simulink library "CockpitDisplayLib"  (R2013b)
settings: Solver=ode45  StartTime=0.0  StopTime=10.0  RelTol=1e-3
undefined symbols (not defined in the file): Ts
libraries: dspadpt3 x3, sf_aircraft_screen_library x1, LandingGearModeLib x1
(part 1 of 2)
settings Model: Creator=siddhars  LastModifiedBy=siddhars

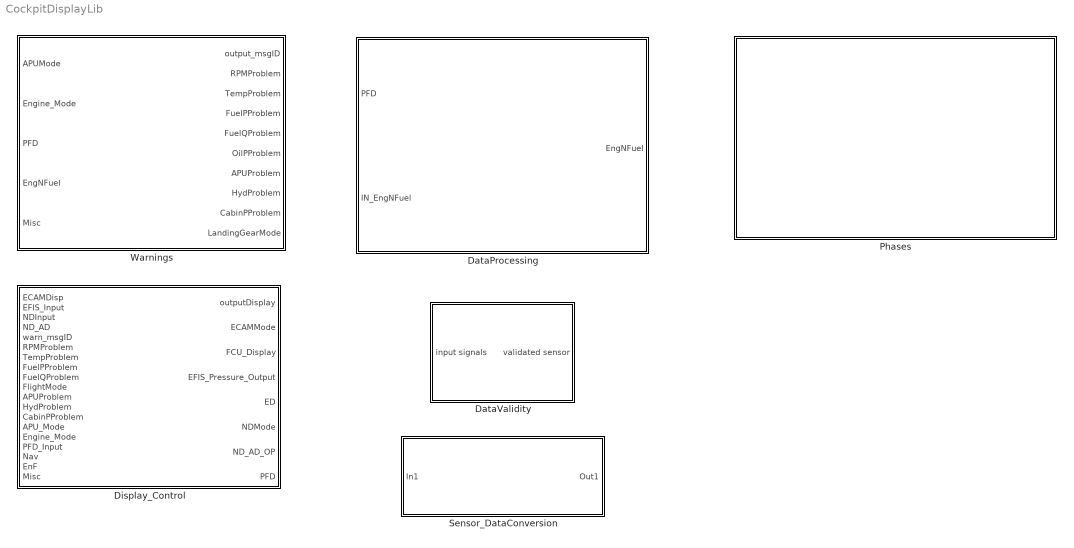
== system CockpitDisplayLib ==
  DataProcessing : Stateflow chart  TreatAsAtomicUnit=on
  DataValidity : Subsystem
  Display_Control : Stateflow chart  TreatAsAtomicUnit=on
  Phases : Stateflow chart  TreatAsAtomicUnit=on
  Sensor_DataConversion : Subsystem  mask{noise_factor=1}
      mask prompts: noise_factor "noise factor"
      mask Callback noise_factor: noise_factor = 1;
  Warnings : Stateflow chart  Priority=0  TreatAsAtomicUnit=on

== system CockpitDisplayLib/DataProcessing/RPMCalc.signal_conditioning ==
  RPM : Inport  OutDataTypeStr=double  PortDimensions=[3 1]
  f : TriggerPort  TriggerType=function-call
      settings: CopyFcn=Stateflow.SLINSF.SimulinkMan.removeBlockPreDeleteFcn  PreDeleteFcn=Stateflow.SLINSF.SimulinkMan.unsafePredeleteFcn
  DataValidity : sf_aircraft_screen_library/Position Monitor, (No Filter)
  Out : Outport
  wires:
  DataValidity/1 -> Out/1
  RPM/1 -> DataValidity/1

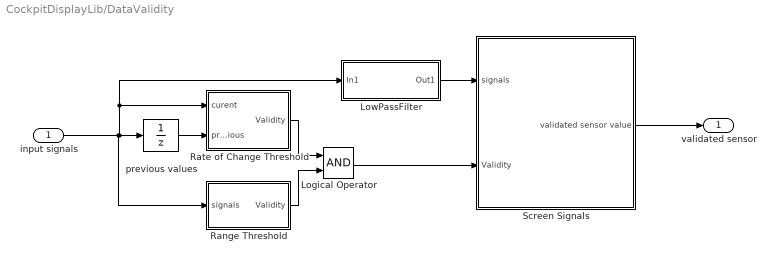
== system CockpitDisplayLib/DataValidity ==
  input signals : Inport  PortDimensions=3
  Logical Operator : Logic  AllPortsSameDT=off
  LowPassFilter : Subsystem
  Range Threshold : Subsystem  RequirementInfo={'other' 'Position Sensor Logic Requirements.doc' 'Out of Bound Readings' 'true' 'Out of Bound Readings' '' } %GIDa_9464ebc1_75a4_4fc1_b22e_333f2b8b1e7f
  Rate of Change Threshold : Subsystem  RequirementInfo={'other' 'Position Sensor Logic Requirements.doc' 'Rate of Change of Readings' 'true' 'Rate of Change of Readings' '' } %GIDa_c48669ac_f48f_472f_ad85_0df61b6d7184  mask{max_rate_change=20000}
      mask prompts: max_rate_change "Rate Change Threshold"
  Screen Signals : Subsystem
  previous values : UnitDelay  SampleTime=-1
  validated sensor : Outport
  wires:
  LowPassFilter/1(Out1) -> Screen Signals/1(signals)
  Screen Signals/1(validated sensor value) -> validated sensor/1
  input signals/1 -> Range Threshold/1(signals), previous values/1, Rate of Change Threshold/1(curent), LowPassFilter/1(In1)
  previous values/1 -> Rate of Change Threshold/2(previous)
  Range Threshold/1(Validity) -> Logical Operator/2
  Rate of Change Threshold/1(Validity) -> Logical Operator/1
  Logical Operator/1 -> Screen Signals/2(Validity)

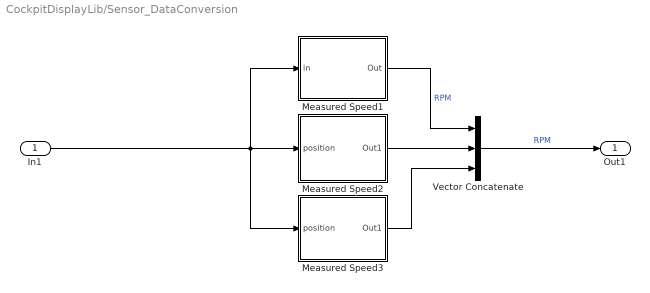
== system CockpitDisplayLib/Sensor_DataConversion ==
  In1 : Inport
  Measured Speed1 : Subsystem
  Measured Speed2 : Subsystem
  Measured Speed3 : Subsystem
  Vector Concatenate : Concatenate  NumInputs=3
  Out1 : Outport
  wires:
  Measured Speed1/1(Out) -> Vector Concatenate/1  "RPM"
  Vector Concatenate/1 -> Out1/1  "RPM"
  Measured Speed3/1(Out1) -> Vector Concatenate/3
  In1/1 -> Measured Speed3/1(position), Measured Speed1/1(in), Measured Speed2/1(position)
  Measured Speed2/1(Out1) -> Vector Concatenate/2

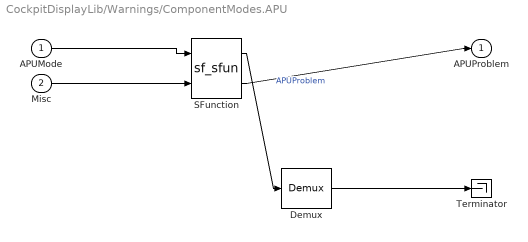
== system CockpitDisplayLib/Warnings/ComponentModes.APU ==
  APUMode : Inport
  Misc : Inport  Port=2
  " Demux " : Demux  Outputs=1
  " SFunction " : S-Function  Tag=Stateflow S-Function CockpitDisplayLib 10  FunctionName=sf_sfun  PortCounts=[2 2]  EnableBusSupport=off
  " Terminator " : Terminator
  APUProblem : Outport
  wires:
  APUMode/1 -> " SFunction "/1
  Misc/1 -> " SFunction "/2
  " SFunction "/2 -> APUProblem/1  "APUProblem"
  " Demux "/1 -> " Terminator "/1
  " SFunction "/1 -> " Demux "/1

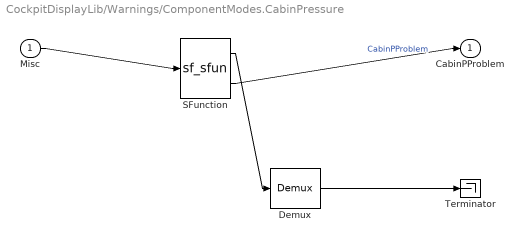
== system CockpitDisplayLib/Warnings/ComponentModes.CabinPressure ==
  Misc : Inport
  " Demux " : Demux  Outputs=1
  " SFunction " : S-Function  Tag=Stateflow S-Function CockpitDisplayLib 11  FunctionName=sf_sfun  PortCounts=[1 2]  EnableBusSupport=off
  " Terminator " : Terminator
  CabinPProblem : Outport
  wires:
  Misc/1 -> " SFunction "/1
  " SFunction "/2 -> CabinPProblem/1  "CabinPProblem"
  " Demux "/1 -> " Terminator "/1
  " SFunction "/1 -> " Demux "/1

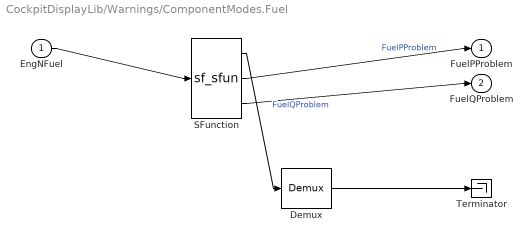
== system CockpitDisplayLib/Warnings/ComponentModes.Fuel ==
  EngNFuel : Inport
  " Demux " : Demux  Outputs=1
  " SFunction " : S-Function  Tag=Stateflow S-Function CockpitDisplayLib 2  FunctionName=sf_sfun  PortCounts=[1 3]  EnableBusSupport=off
  " Terminator " : Terminator
  FuelPProblem : Outport
  FuelQProblem : Outport  Port=2
  wires:
  EngNFuel/1 -> " SFunction "/1
  " SFunction "/2 -> FuelPProblem/1  "FuelPProblem"
  " SFunction "/3 -> FuelQProblem/1  "FuelQProblem"
  " Demux "/1 -> " Terminator "/1
  " SFunction "/1 -> " Demux "/1

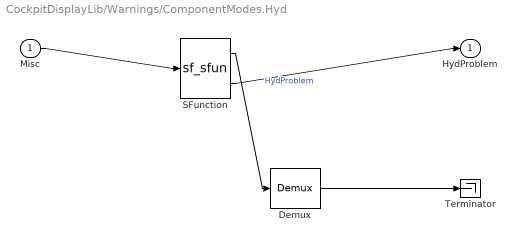
== system CockpitDisplayLib/Warnings/ComponentModes.Hyd ==
  Misc : Inport
  " Demux " : Demux  Outputs=1
  " SFunction " : S-Function  Tag=Stateflow S-Function CockpitDisplayLib 13  FunctionName=sf_sfun  PortCounts=[1 2]  EnableBusSupport=off
  " Terminator " : Terminator
  HydProblem : Outport
  wires:
  Misc/1 -> " SFunction "/1
  " SFunction "/2 -> HydProblem/1  "HydProblem"
  " Demux "/1 -> " Terminator "/1
  " SFunction "/1 -> " Demux "/1

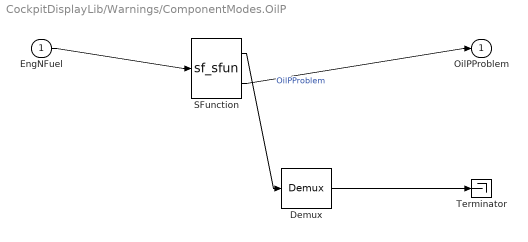
== system CockpitDisplayLib/Warnings/ComponentModes.OilP ==
  EngNFuel : Inport
  " Demux " : Demux  Outputs=1
  " SFunction " : S-Function  Tag=Stateflow S-Function CockpitDisplayLib 15  FunctionName=sf_sfun  PortCounts=[1 2]  EnableBusSupport=off
  " Terminator " : Terminator
  OilPProblem : Outport
  wires:
  EngNFuel/1 -> " SFunction "/1
  " SFunction "/2 -> OilPProblem/1  "OilPProblem"
  " Demux "/1 -> " Terminator "/1
  " SFunction "/1 -> " Demux "/1

== system CockpitDisplayLib/Warnings/ComponentModes.RPM ==
  EngNFuel : Inport
  " Demux " : Demux  Outputs=1
  " SFunction " : S-Function  Tag=Stateflow S-Function CockpitDisplayLib 16  FunctionName=sf_sfun  PortCounts=[1 2]  EnableBusSupport=off
  " Terminator " : Terminator
  RPMProblem : Outport
  wires:
  EngNFuel/1 -> " SFunction "/1
  " SFunction "/2 -> RPMProblem/1  "RPMProblem"
  " Demux "/1 -> " Terminator "/1
  " SFunction "/1 -> " Demux "/1

== system CockpitDisplayLib/Warnings/ComponentModes.Temp ==
  EngNFuel : Inport
  " Demux " : Demux  Outputs=1
  " SFunction " : S-Function  Tag=Stateflow S-Function CockpitDisplayLib 17  FunctionName=sf_sfun  PortCounts=[1 2]  EnableBusSupport=off
  " Terminator " : Terminator
  TempProblem : Outport
  wires:
  EngNFuel/1 -> " SFunction "/1
  " SFunction "/2 -> TempProblem/1  "TempProblem"
  " Demux "/1 -> " Terminator "/1
  " SFunction "/1 -> " Demux "/1

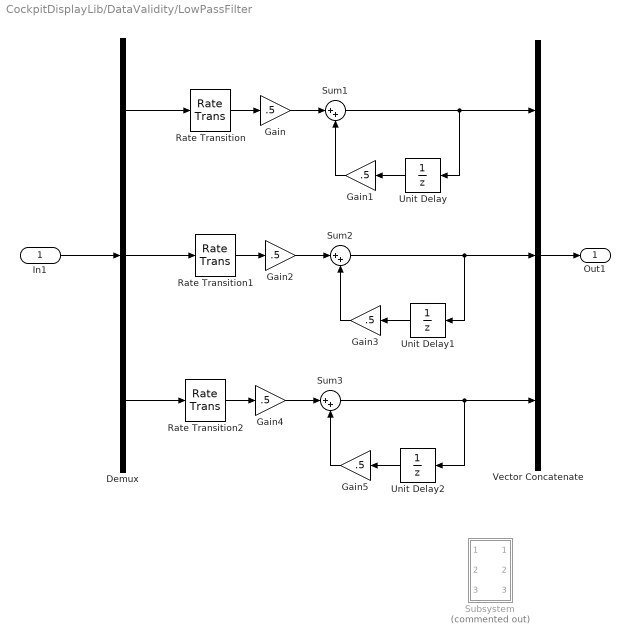
== system CockpitDisplayLib/DataValidity/LowPassFilter ==
  In1 : Inport
  Demux : Demux  Outputs=3
  Gain{,1..5} (6 alike) : Gain  Gain=.5
  Rate Transition : RateTransition
  Rate Transition1 : RateTransition
  Rate Transition2 : RateTransition
  Subsystem : Subsystem  Commented=on
  Sum1 : Sum  Inputs=|++
  Sum2 : Sum  Inputs=|++
  Sum3 : Sum  Inputs=|++
  Unit Delay : UnitDelay  SampleTime=-1
  Unit Delay1 : UnitDelay  SampleTime=-1
  Unit Delay2 : UnitDelay  SampleTime=-1
  Vector Concatenate : Concatenate  NumInputs=3
  Out1 : Outport
  wires:
  Rate Transition2/1 -> Gain4/1
  Gain5/1 -> Sum3/2
  Unit Delay2/1 -> Gain5/1
  Gain4/1 -> Sum3/1
  Demux/3 -> Rate Transition2/1
  Sum3/1 -> Unit Delay2/1, Vector Concatenate/3
  Rate Transition1/1 -> Gain2/1
  Gain3/1 -> Sum2/2
  Unit Delay1/1 -> Gain3/1
  Gain2/1 -> Sum2/1
  Demux/2 -> Rate Transition1/1
  Sum2/1 -> Unit Delay1/1, Vector Concatenate/2
  Rate Transition/1 -> Gain/1
  Gain1/1 -> Sum1/2
  Unit Delay/1 -> Gain1/1
  Gain/1 -> Sum1/1
  Demux/1 -> Rate Transition/1
  Sum1/1 -> Vector Concatenate/1, Unit Delay/1
  In1/1 -> Demux/1
  Vector Concatenate/1 -> Out1/1

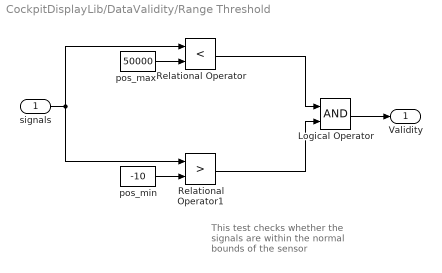
== system CockpitDisplayLib/DataValidity/Range Threshold ==
  note: This test checks whether the signals are within
      | the normal bounds of the sensor
  signals : Inport
  Logical Operator : Logic  AllPortsSameDT=off
  Relational Operator : RelationalOperator  Operator=<
  Relational Operator1 : RelationalOperator  Operator=>
  pos_max : Constant  Value=50000
  pos_min : Constant  Value=-10
  Validity : Outport
  wires:
  Logical Operator/1 -> Validity/1
  pos_min/1 -> Relational Operator1/2
  pos_max/1 -> Relational Operator/2
  Relational Operator1/1 -> Logical Operator/2
  Relational Operator/1 -> Logical Operator/1
  signals/1 -> Relational Operator1/1, Relational Operator/1

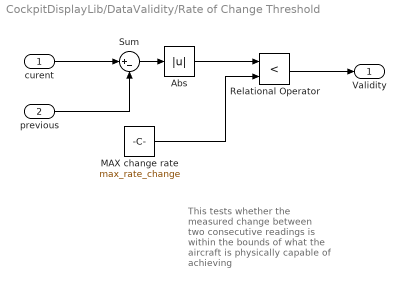
== system CockpitDisplayLib/DataValidity/Rate of Change Threshold ==
  note: This tests whether the measured change between two consecutive readings
      | is within the bounds of what the aircraft is physically capable of achieving
  curent : Inport
  previous : Inport  Port=2
  Abs : Abs  SaturateOnIntegerOverflow=on
  MAX change rate : Constant  Value=max_rate_change
  Relational Operator : RelationalOperator  Operator=<  OutDataTypeStr=boolean
  Sum : Sum  Inputs=|+-  SaturateOnIntegerOverflow=on
  Validity : Outport
  wires:
  curent/1 -> Sum/1
  previous/1 -> Sum/2
  Relational Operator/1 -> Validity/1
  MAX change rate/1 -> Relational Operator/2
  Sum/1 -> Abs/1
  Abs/1 -> Relational Operator/1

== system CockpitDisplayLib/DataValidity/Screen Signals ==
  signals : Inport
  Validity : Inport  Port=2
  Chart (MATLAB) : Stateflow chart  TreatAsAtomicUnit=on
  Data Type Conversion : DataTypeConversion  OutDataTypeStr=double
  validated sensor value : Outport
  wires:
  Chart (MATLAB)/1(valid_signal) -> validated sensor value/1
  Validity/1 -> Data Type Conversion/1
  signals/1 -> Chart (MATLAB)/1(signals)
  Data Type Conversion/1 -> Chart (MATLAB)/2(validity)

== system CockpitDisplayLib/Sensor_DataConversion/Measured Speed1 ==
  in : Inport
  Random Number : RandomNumber  Variance=.001*noise_factor  SampleTime=Ts
  Sum1 : Sum  Inputs=|++  SaturateOnIntegerOverflow=on
  Out : Outport
  wires:
  Sum1/1 -> Out/1
  in/1 -> Sum1/1
  Random Number/1 -> Sum1/2

== system CockpitDisplayLib/Sensor_DataConversion/Measured Speed2 ==
  position : Inport
  Random Number : RandomNumber  Variance=.001*noise_factor  SampleTime=Ts
  Sum1 : Sum  Inputs=|++  SaturateOnIntegerOverflow=on
  Out1 : Outport
  wires:
  Random Number/1 -> Sum1/2
  position/1 -> Sum1/1
  Sum1/1 -> Out1/1

== system CockpitDisplayLib/Sensor_DataConversion/Measured Speed3 ==
  position : Inport
  Random Number : RandomNumber  Variance=.001*noise_factor  SampleTime=Ts
  Sum : Sum  Inputs=|++  SaturateOnIntegerOverflow=on
  Out1 : Outport
  wires:
  Sum/1 -> Out1/1
  position/1 -> Sum/1
  Random Number/1 -> Sum/2

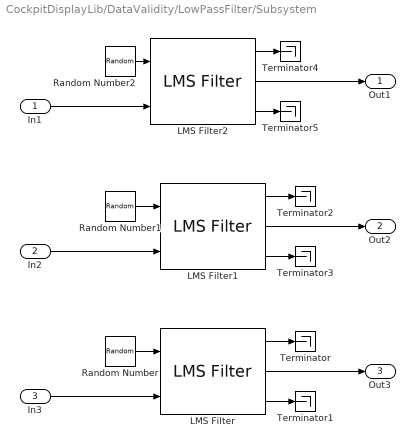
== system CockpitDisplayLib/DataValidity/LowPassFilter/Subsystem ==
  In1 : Inport
  In2 : Inport  Port=2
  In3 : Inport  Port=3
  LMS Filter : dspadpt3/LMS Filter  Algo=LMS  L=2  stepflag=Dialog  mu=0.1  leakage=1.0  ic=0  Adapt=off  resetflag=None  weights=on  secondCoeffMode=User-defined  secondCoeffWordLength=2  secondCoeffFracLength=15  accum2Mode=User-defined  accum2FracLength=20  prodOutput2Mode=User-defined  prodOutput2FracLength=20  prodOutput3Mode=User-defined  prodOutput3FracLength=20  prodOutput4Mode=User-defined  prodOutput4FracLength=20  quotientMode=User-defined  quotientFracLength=20  roundingMode=Floor  overflowMode=off  addnparflag=off
  LMS Filter1 : dspadpt3/LMS Filter  Algo=LMS  L=2  stepflag=Dialog  mu=0.1  leakage=1.0  ic=0  Adapt=off  resetflag=None  weights=on  secondCoeffMode=User-defined  secondCoeffWordLength=2  secondCoeffFracLength=15  accum2Mode=User-defined  accum2FracLength=20  prodOutput2Mode=User-defined  prodOutput2FracLength=20  prodOutput3Mode=User-defined  prodOutput3FracLength=20  prodOutput4Mode=User-defined  prodOutput4FracLength=20  quotientMode=User-defined  quotientFracLength=20  roundingMode=Floor  overflowMode=off  addnparflag=off
  LMS Filter2 : dspadpt3/LMS Filter  Algo=LMS  L=2  stepflag=Dialog  mu=0.1  leakage=1.0  ic=0  Adapt=off  resetflag=None  weights=on  secondCoeffMode=User-defined  secondCoeffWordLength=2  secondCoeffFracLength=15  accum2Mode=User-defined  accum2FracLength=20  prodOutput2Mode=User-defined  prodOutput2FracLength=20  prodOutput3Mode=User-defined  prodOutput3FracLength=20  prodOutput4Mode=User-defined  prodOutput4FracLength=20  quotientMode=User-defined  quotientFracLength=20  roundingMode=Floor  overflowMode=off  addnparflag=off
  Random Number : RandomNumber  Variance=0.01  SampleTime=Ts
  Random Number1 : RandomNumber  Variance=0.01  SampleTime=Ts
  Random Number2 : RandomNumber  Variance=0.01  SampleTime=Ts
  Terminator{,1..5} (6 alike) : Terminator
  Out1 : Outport
  Out2 : Outport  Port=2
  Out3 : Outport  Port=3
  wires:
  LMS Filter2/1 -> Terminator4/1
  LMS Filter2/3 -> Terminator5/1
  Random Number2/1 -> LMS Filter2/1
  LMS Filter1/1 -> Terminator2/1
  Random Number1/1 -> LMS Filter1/1
  LMS Filter/3 -> Terminator1/1
  LMS Filter1/3 -> Terminator3/1
  LMS Filter/2 -> Out3/1
  LMS Filter2/2 -> Out1/1
  In1/1 -> LMS Filter2/2
  In3/1 -> LMS Filter/2
  In2/1 -> LMS Filter1/2
  LMS Filter1/2 -> Out2/1
  Random Number/1 -> LMS Filter/1
  LMS Filter/1 -> Terminator/1

== stateflow chart CockpitDisplayLib/Display_Control ==
  state PrimaryFlightDisplay [parallel]
    entry, during:
    PFD.AirSpeed = PFD_Input.AirSpeed;
    PFD.Attitude = PFD_Input.Attitude;
    PFD.Heading = PFD_Input.Direction;
    PFD.Altitude = PFD_Input.Altitude;
    settings: executionOrder=1
    state AirSpeed [parallel]
      settings: executionOrder=1
      state Starting
        entry:
        PFD.AirSpeedMode = -1;
      state OFF
      state Running
        entry: PFD.AirSpeedMode = 1;
      (default) -> PrimaryFlightDisplay.AirSpeed.OFF
      PrimaryFlightDisplay.AirSpeed.OFF -> PrimaryFlightDisplay.AirSpeed.Starting : [APU_Mode  == 1]
      PrimaryFlightDisplay.AirSpeed.Starting -> PrimaryFlightDisplay.AirSpeed.Running : after(5,sec)
    state Altitude [parallel]
      settings: executionOrder=2
      state OFF
      state Starting
        entry:
        PFD.AltMode = -1;
      state Running
        entry: PFD.AltMode = 1;
      (default) -> PrimaryFlightDisplay.Altitude.OFF
      PrimaryFlightDisplay.Altitude.OFF -> PrimaryFlightDisplay.Altitude.Starting : [APU_Mode  == 1]
      PrimaryFlightDisplay.Altitude.Starting -> PrimaryFlightDisplay.Altitude.Running : after(5,sec)
    state Heading [parallel]
      settings: executionOrder=3
      state OFF
      state Starting
        entry:
        PFD.HeadingMode = -1;
      state Running
        entry: PFD.HeadingMode = 1;
      (default) -> PrimaryFlightDisplay.Heading.OFF
      PrimaryFlightDisplay.Heading.OFF -> PrimaryFlightDisplay.Heading.Starting : [APU_Mode  == 1]
      PrimaryFlightDisplay.Heading.Starting -> PrimaryFlightDisplay.Heading.Running : after(5,sec)
    state Attitude [parallel]
      settings: executionOrder=4
      state OFF
      state Starting
        entry:
        PFD.AttMode = -1;
      state Running
        entry: PFD.AttMode = 1;
      (default) -> PrimaryFlightDisplay.Attitude.OFF
      PrimaryFlightDisplay.Attitude.OFF -> PrimaryFlightDisplay.Attitude.Starting : [APU_Mode  == 1]
      PrimaryFlightDisplay.Attitude.Starting -> PrimaryFlightDisplay.Attitude.Running : after(5,sec)
  state NavigationDisplay [parallel]
    settings: executionOrder=2
    state NDDisplayPages [parallel]
      settings: executionOrder=1
      state NDRunning
        state ILSPage
          entry:
          NDMode = 1;
        state VORPage
          entry:
          NDMode = 2;
        state NAVPage
          entry:
          NDMode = 3;
        state ARCPage
          entry:
          NDMode = 4;
        state PLANPage
          entry:
          NDMode = 5;
        NDRunning -> (junction 257)
        (junction 257) -> ILSPage [order 1] : [NDInput == NDPageInput.ILS]
        (junction 257) -> PLANPage [order 5] : [NDInput == NDPageInput.PLAN]
        (junction 257) -> VORPage [order 2] : [NDInput == NDPageInput.VOR]
        (junction 257) -> ARCPage [order 4] : [NDInput == NDPageInput.ARC]
        (junction 257) -> NAVPage [order 3] : [NDInput == NDPageInput.NAV]
      state NDOff
      state NDStart
        entry:
        NDMode = -1;
      (default) -> NDOff
      NDOff -> NDStart : [APU_Mode  == 1]
      NDStart -> ILSPage : after(3,sec)
    state CSTRDisplay [parallel]
      settings: executionOrder=2
      state OFF
        entry:
        ND_AD_OP.CSTR=0;
      state ON
        entry:
        ND_AD_OP.CSTR=1;
      (default) -> NavigationDisplay.CSTRDisplay.OFF
      NavigationDisplay.CSTRDisplay.OFF -> NavigationDisplay.CSTRDisplay.ON : [ND_AD.CSTR==1&& in(NDDisplayPages.NDRunning)]
      NavigationDisplay.CSTRDisplay.ON -> NavigationDisplay.CSTRDisplay.OFF : [ND_AD.CSTR==0]
    state WPTDisplay [parallel]
      settings: executionOrder=3
      state OFF
        entry:
        ND_AD_OP.WPT=0;
      state ON
        entry:
        ND_AD_OP.WPT=1;
      (default) -> NavigationDisplay.WPTDisplay.OFF
      NavigationDisplay.WPTDisplay.OFF -> NavigationDisplay.WPTDisplay.ON : [ND_AD.WPT==1&& in(NDDisplayPages.NDRunning)]
      NavigationDisplay.WPTDisplay.ON -> NavigationDisplay.WPTDisplay.OFF : [ND_AD.WPT==0]
    state VORDDisplay [parallel]
      settings: executionOrder=4
      state OFF
        entry:
        ND_AD_OP.VORD= 0;
      state ON
        entry:
        ND_AD_OP.VORD= 1;
      (default) -> NavigationDisplay.VORDDisplay.OFF
      NavigationDisplay.VORDDisplay.OFF -> NavigationDisplay.VORDDisplay.ON : [ND_AD.VORD==1&& in(NDDisplayPages.NDRunning)]
      NavigationDisplay.VORDDisplay.ON -> NavigationDisplay.VORDDisplay.OFF : [ND_AD.VORD==0]
    state NDBDisplay [parallel]
      settings: executionOrder=5
      state OFF
        entry:
        ND_AD_OP.NDB= 0;
      state ON
        entry:
        ND_AD_OP.NDB= 1;
      (default) -> NavigationDisplay.NDBDisplay.OFF
      NavigationDisplay.NDBDisplay.OFF -> NavigationDisplay.NDBDisplay.ON : [ND_AD.NDB==1&& in(NDDisplayPages.NDRunning)]
      NavigationDisplay.NDBDisplay.ON -> NavigationDisplay.NDBDisplay.OFF : [ND_AD.NDB==0]
    state ARPTDisplay [parallel]
      settings: executionOrder=6
      state OFF
        entry:
        ND_AD_OP.ARPT= 0;
      state ON
        entry:
        ND_AD_OP.ARPT= 1;
      (default) -> NavigationDisplay.ARPTDisplay.OFF
      NavigationDisplay.ARPTDisplay.OFF -> NavigationDisplay.ARPTDisplay.ON : [ND_AD.ARPT==1&& in(NDDisplayPages.NDRunning)]
      NavigationDisplay.ARPTDisplay.ON -> NavigationDisplay.ARPTDisplay.OFF : [ND_AD.ARPT==0]
  state EngineDisplay [parallel]
    entry, during:
    outputDisplay.warn_msgID = warn_msgID;
    outputDisplay.flightmode = FlightMode;
    ED.N1_L = EnF.RPM;
    ED.N1_R = EnF.RPM;
    ED.FlapConfig = calcFlapConfig(FlightMode);
    ED.EGT1 = EnF.EGT;
    ED.EGT2 = EnF.EGT;
    ED.EPR1 = EnF.EPR1;
    ED.EPR2 = EnF.EPR2;
    ED.FuelQuantity = EnF.FuelQuantity;
    settings: executionOrder=3
    state out = calcFlapConfig(flightphase) [function]
      (default) -> (junction 230) : % comment
      (junction 230) -> (junction 233) [order 1] : [flightphase == 1]
      (junction 230) -> (junction 232) [order 2]
      (junction 233) -> (junction 234) : {out = 1;}
      (junction 232) -> (junction 235) [order 1] : [flightphase == 2]
      (junction 232) -> (junction 231) [order 2] : {out = 3;}
      (junction 235) -> (junction 236) : {out = 2;}
      (junction 236) -> (junction 231)
      (junction 234) -> (junction 236)
      (junction 231) -> (junction 237)
    state Engine_Running
      entry, during:
      ED.ED_Mode_L = 1;
      ED.ED_Mode_R = 1;
      outputDisplay.ED_Mode_L = 1;
      outputDisplay.ED_Mode_R = 1;
    state Engine_Ready
      entry, during:
      ED.ED_Mode_L = 1;
      ED.ED_Mode_R = 1;
      outputDisplay.ED_Mode_L = 1;
      outputDisplay.ED_Mode_R = 1;
    state Engine_Off
    state Engine_Boot
      entry, during:
      ED.ED_Mode_L = -1;
      ED.ED_Mode_R = -1;
      outputDisplay.ED_Mode_L = -1;
      outputDisplay.ED_Mode_R = -1;
    (default) -> Engine_Off
    Engine_Ready -> Engine_Running : [Engine_Mode == 2]
    Engine_Boot -> Engine_Ready : after(5,sec)
    Engine_Off -> Engine_Boot : [Engine_Mode == 1]
  state FCU_EFIS_Display [parallel]
    entry, during:
    FCU_Display.Speed =  PFD_Input.AirSpeed;
    FCU_Display.Heading = Nav.selectedheading;
    FCU_Display.Altitude = PFD_Input.Altitude;
    if EFIS_Input == EFIS_Pressure.inHg
    EFIS_Pressure_Output = Misc.CabinPressure;
    else
    EFIS_Pressure_Output = Misc.CabinPressure*25.4;
    end
    settings: executionOrder=5
  state SystemDisplay [parallel]
    settings: executionOrder=4
    state Startup
      state APU_Ready
        entry:
        ECAMMode = 8;
      state APU_Running
        entry:
        ECAMMode = 8;
      state APU_Boot
        entry:
        ECAMMode = -1;
      state APU_Off
      state APU_Wait
        entry:
        ECAMMode = 11 ;
      state EngineStarting
        entry:
        ECAMMode = 4 ;
      (default) -> APU_Off
      APU_Off -> APU_Boot : [APU_Mode  == 1]
      APU_Boot -> APU_Ready : after(2,sec)
      APU_Ready -> APU_Running : [APU_Mode == 2]
      APU_Wait -> EngineStarting : [Engine_Mode == 1]
      APU_Running -> APU_Wait : after(3,sec)
    state NormalFlight
      state PushbackAndTaxi
        entry: ECAMMode = 1;
      state TakeoffCruiseDescent
        entry: ECAMMode = 2;
      state Land
        entry: ECAMMode = 3;
      NormalFlight -> (junction 92) [order 1]
      (default) -> (junction 92)
      (junction 92) -> PushbackAndTaxi [order 1] : [FlightMode == 1]
      (junction 92) -> Land [order 3]
      (junction 92) -> TakeoffCruiseDescent [order 2] : [FlightMode == 2]
    state UserSelection_Faults
      state Engine
        entry:
        ECAMMode = 4;
      state Cabin_Pressure
        entry:
        ECAMMode = 10;
      state HYD
        entry:
        ECAMMode = 7;
      state FUEL
        entry:
        ECAMMode = 9;
      state APU
        entry:
        ECAMMode = 8;
      state Bleed
        entry:
        ECAMMode = 5;
      state ERROR
      (default) -> (junction 380)
      (junction 380) -> (junction 385) [order 1] : [ECAMDisp~= 0]
      (junction 380) -> (junction 386) [order 2]
      (junction 385) -> (junction 373)
      (junction 386) -> (junction 78)
      (junction 373) -> Engine [order 1] : [ECAMDisp == ECAMInput.ENG]
      (junction 78) -> Engine [order 1] : [RPMProblem >0||TempProblem > 0]
      (junction 373) -> (junction 366) [order 2]
      (junction 78) -> (junction 389) [order 2]
      Engine -> UserSelection_Faults : after(5,sec)
      (junction 366) -> Cabin_Pressure [order 1] : [ECAMDisp == ECAMInput.PRESS]
      (junction 389) -> Cabin_Pressure [order 1] : [CabinPProblem > 0]
      (junction 366) -> (junction 364) [order 2]
      (junction 389) -> (junction 136) [order 2]
      Cabin_Pressure -> UserSelection_Faults : after(5,sec)
      (junction 136) -> HYD [order 1] : [HydProblem > 0]
      (junction 364) -> HYD [order 1] : [ECAMDisp == ECAMInput.HYD]
      (junction 136) -> (junction 137) [order 2]
      (junction 364) -> (junction 375) [order 2]
      HYD -> UserSelection_Faults : after(5,sec)
      (junction 137) -> FUEL [order 1] : [FuelPProblem > 0 || ...
          | FuelQProblem > 0]
      (junction 137) -> (junction 138) [order 2]
      (junction 375) -> FUEL [order 1] : [ECAMDisp == ECAMInput.FUEL]
      (junction 375) -> (junction 377) [order 2]
      FUEL -> UserSelection_Faults : after(5,sec)
      (junction 138) -> APU [order 1] : [APUProblem > 0]
      (junction 377) -> APU [order 1] : [ECAMDisp == ECAMInput.APU]
      (junction 138) -> (junction 352) [order 2]
      (junction 377) -> (junction 357) [order 2]
      APU -> UserSelection_Faults : after(5,sec)
      (junction 357) -> Bleed : [ECAMDisp == ECAMInput.BLEED]
      Bleed -> UserSelection_Faults : after(5,sec)
      (junction 352) -> ERROR
    (default) -> Startup
    EngineStarting -> NormalFlight : [FlightMode > 0]
    UserSelection_Faults -> NormalFlight : after(1,sec)[all([RPMProblem, TempProblem,...
        | HydProblem, APUProblem, FuelPProblem,...
        | FuelQProblem,CabinPProblem]==0) &&...
        | (ECAMDisp==0)]
    NormalFlight -> UserSelection_Faults [order 1] : [any([RPMProblem, TempProblem,HydProblem,...
        |  APUProblem, FuelPProblem,FuelQProblem,...
        | CabinPProblem]~=0)||...
        |  ECAMDisp~=0]
  data: flightphase function_input; out function_output; ECAMDisp input; EFIS_Input input; NDInput input; ND_AD input Bus: NDAdditionalDisplay; warn_msgID input; outputDisplay output Bus: warnings_bus; RPMProblem input; TempProblem input; FuelPProblem input; FuelQProblem input; FlightMode input; APUProblem input; HydProblem input; CabinPProblem input; APU_Mode input; Engine_Mode input; PFD_Input input Bus: FlightInputs; Nav input Bus: NavData; ECAMMode output double; FCU_Display output Bus: FCU_Output; EnF input Bus: EngineFuel_Bus; Misc input Bus: MiscData; EFIS_Pressure_Output output; ED output Bus: EngineDisplayBus; NDMode output; ND_AD_OP output Bus: NDAdditionalDisplay; PFD output Bus: PFDOutput

== stateflow chart CockpitDisplayLib/Warnings/ComponentModes.Fuel ==
  state FuelPressureModes [parallel]
    settings: executionOrder=1
    state Normal
      entry:
      FuelPProblem = 0;
    state FuelPressureLow
      entry:
      FuelPProblem = 1;
    (default) -> FuelPressureModes.Normal
    FuelPressureModes.Normal -> FuelPressureLow : [funcFuelPressLow()]
    FuelPressureLow -> FuelPressureModes.Normal : [~funcFuelPressLow()]
  state FuelQuantityModes [parallel]
    settings: executionOrder=2
    state Normal
      entry:
      FuelQProblem = 0;
    state FuelQuantityLow
      entry:
      FuelQProblem = 1;
    (default) -> FuelQuantityModes.Normal
    FuelQuantityLow -> FuelQuantityModes.Normal : [~funcFuelQuantityLow()]
    FuelQuantityModes.Normal -> FuelQuantityLow : [funcFuelQuantityLow()]
  state y = funcFuelQuantityLow [function]
    (default) -> (junction 47) : {y = 0;}
    (junction 47) -> (junction 48) [order 1] : [FlightMode == 1]
    (junction 48) -> (junction 49) : [EngNFuel.FuelQuantity<20000]
    (junction 47) -> (junction 50) [order 2]
    (junction 49) -> (junction 52)
    (junction 50) -> (junction 51) [order 1] : [FlightMode == 2]
    (junction 51) -> (junction 52) : [EngNFuel.FuelQuantity<10000]
    (junction 50) -> (junction 53) [order 2] : {y = 0;}
    (junction 52) -> (junction 54) : {y = 1;}
    (junction 53) -> (junction 54)
  state y = funcFuelPressLow [function]
    (default) -> (junction 16) : {y = 0;}
    (junction 16) -> (junction 17) [order 1] : [FlightMode == 1]
    (junction 17) -> (junction 18) : [EngNFuel.fuelpressure<5]
    (junction 16) -> (junction 19) [order 2]
    (junction 18) -> (junction 26)
    (junction 19) -> (junction 20) [order 1] : [FlightMode == 2]
    (junction 19) -> (junction 21) [order 2]
    (junction 20) -> (junction 24)
    (junction 21) -> (junction 22) : [FlightMode == 3]
    (junction 22) -> (junction 23)
    (junction 23) -> (junction 24)
    (junction 24) -> (junction 25)
    (junction 25) -> (junction 26) [order 1] : [EngNFuel.fuelpressure<15]
    (junction 25) -> (junction 27) [order 2] : {y = 0;}
    (junction 26) -> (junction 28) : {y = 1;}
    (junction 27) -> (junction 28)
  data: y function_output double size=1; y function_output double size=1; EngNFuel input Bus: EngineFuel_Bus; FuelPProblem output double size=1; FuelQProblem output double size=1; FlightMode data_store_memory size=1

== stateflow chart CockpitDisplayLib/Phases ==
  state Ph1
  state Ph2
  state Ph3
  state Ph4
  state Ph5
  state Ph6
  state Ph7
  state Ph8
  state Ph9
  state Ph10
  state End
  (default) -> Ph1 : % start electric power
  Ph1 -> Ph2 : % 1st engine started
  Ph2 -> Ph3 : % 1st engine T.O. power
  Ph3 -> Ph4 : % 80 kts
  Ph4 -> Ph5 : % lift off
  Ph5 -> Ph6 : % 1600 ft
  Ph6 -> Ph7 : % 800 ft
  Ph7 -> Ph8 : % touch down
  Ph8 -> Ph9 : % 80 kts
  Ph9 -> Ph10 : % 2nd engine SHUT ON
  Ph10 -> End : after(5,sec)

== stateflow chart CockpitDisplayLib/DataProcessing ==
  state RPMCalc [parallel]
    entry, during:
    EngNFuel.RPM = signal_conditioning(IN_EngNFuel.RPM);
    settings: executionOrder=1
    state Out = signal_conditioning(RPM) [function]
  state TemperatureCalc [parallel]
    settings: executionOrder=2
  state FuelFlowCalc [parallel]
    settings: executionOrder=3
  state OilPressureCalc [parallel]
    settings: executionOrder=4
  state BearingCalc [parallel]
    settings: executionOrder=5
  state GroundspeedCalc [parallel]
    settings: executionOrder=7
  state SelectedHeadingCalc [parallel]
    settings: executionOrder=8
  state DistanceCalc [parallel]
    settings: executionOrder=6
  state RateOfTurnCalc [parallel]
    settings: executionOrder=9
  state VerticalSpeedCalc [parallel]
    settings: executionOrder=10
  state DIRECTIONCalc [parallel]
    settings: executionOrder=11
  state ALTITUDECalc [parallel]
    settings: executionOrder=12
  state AirspeedCalc [parallel]
    settings: executionOrder=13
  state ATTITUDECalc [parallel]
    settings: executionOrder=14
  data: RPM function_input double size=[3 1]; Out function_output; PFD input; IN_EngNFuel input Bus: IN_EngineFuel_Bus; EngNFuel output Bus: EngineFuel_Bus

== stateflow chart CockpitDisplayLib/DataValidity/Screen Signals/Chart (MATLAB) ==
  state Screen
    note: no valid signals
    state three
      (default) -> (junction 112) : {sum_sig=signals(1)+signals(2)+signals(3);}
      (junction 112) -> (junction 114) : {middle=sum_sig - (max(signals) + min(signals));}
      (junction 114) -> (junction 113) [order 1] : [bad==1]
      (junction 113) -> (junction 116) : {none();}
      (junction 114) -> (junction 115) [order 2] : {valid_signal=middle;}
      (junction 115) -> (junction 117)
      (junction 117) -> (junction 118) : {prev_signal=valid_signal;}
      (junction 118) -> (junction 119) : {count=0;}
    state zero
      (default) -> (junction 129) : {none();}
    state one
      note: Only one valid sensor - just use the valid signal.
          | Failure is false
      (default) -> (junction 102) : {valid_signal=signals(select(1));}
      (junction 102) -> (junction 103) : {prev_signal=valid_signal;}
      (junction 103) -> (junction 104) : {count=0;}
    state two
      (default) -> (junction 24) : {diff=abs(signals(select(1))-signals(select(2)));}
      (junction 24) -> (junction 23) [order 1] : [diff>diff_max]
      (junction 23) -> (junction 26) : {none();}
      (junction 24) -> (junction 25) [order 2] : {mean=(signals(select(1))+signals(select(2)))/2;}
      (junction 25) -> (junction 27) : {valid_signal=mean;}
      (junction 27) -> (junction 28) : {prev_signal=valid_signal;}
      (junction 28) -> (junction 29) : {count=0;}
    (default) -> (junction 131) : {n=valid_sensors();bad = 0;}
    three -> Screen
    (junction 131) -> zero [order 4]
    (junction 131) -> three [order 1] : [n==3]
    zero -> Screen
    (junction 131) -> two [order 2] : [n==2]
    (junction 131) -> one [order 3] : [n==1]
    one -> Screen
    two -> Screen
  state none [function]
    (default) -> (junction 2)
    (junction 2) -> (junction 3) : {count=count+1;}
    (junction 3) -> (junction 4) [order 1] : [count>3]
    (junction 4) -> (junction 5) : {count=3;}
    (junction 5) -> (junction 6) : {valid_signal=0;}
    (junction 3) -> (junction 7) [order 2] : {valid_signal=prev_signal;}
    (junction 6) -> (junction 9)
    (junction 7) -> (junction 8)
    (junction 8) -> (junction 9)
  (default) -> Screen : {bad = 0;count = 0;prev_signal = 0;}
  data: middle local double; diff local double; mean local double; num function_output double size=1; signals input double size=3; prev_signal local double size=1; count local double size=1; diff_max constant double =3; bad local double size=1; validity input; valid_signal output; sum_sig local double size=1; n local; select local double size=2
  function num = valid_sensors:
    | function num = valid_sensors
    | 
    | aVarTruthTableCondition_1 = false;
    | aVarTruthTableCondition_2 = false;
    | aVarTruthTableCondition_3 = false;
    | 
    | 
    | 
    | aVarTruthTableCondition_1 = logical(validity(1) == 1);
    | 
    | 
    | aVarTruthTableCondition_2 = logical(validity(2) == 1);
    | 
    | 
    | aVarTruthTableCondition_3 = logical(validity(3) == 1);
    | 
    | if (aVarTruthTableCondition_1 && aVarTruthTableCondition_2 && aVarTruthTableCondition_3)
    |     aFcnTruthTableAction_1();
    | elseif (aVarTruthTableCondition_1 && aVarTruthTableCondition_2 && ~aVarTruthTableCondition_3)
    |     aFcnTruthTableAction_2();
    | elseif (aVarTruthTableCondition_1 && ~aVarTruthTableCondition_2 && aVarTruthTableCondition_3)
    |     aFcnTruthTableAction_3();
    | elseif (aVarTruthTableCondition_1 && ~aVarTruthTableCondition_2 && ~aVarTruthTableCondition_3)
    |     aFcnTruthTableAction_5();
    | elseif (~aVarTruthTableCondition_1 && aVarTruthTableCondition_2 && aVarTruthTableCondition_3)
    |     aFcnTruthTableAction_4();
    | elseif (~aVarTruthTableCondition_1 && aVarTruthTableCondition_2 && ~aVarTruthTableCondition_3)
    |     aFcnTruthTableAction_6();
    | elseif (~aVarTruthTableCondition_1 && ~aVarTruthTableCondition_2 && aVarTruthTableCondition_3)
    |     aFcnTruthTableAction_7();
    | else % Default
    |     None();
    | end
    | 
    | function aFcnTruthTableAction_1()
    | 
    | % All 3 signals valid
    | 
    | num = 3;
    | 
    | function aFcnTruthTableAction_2()
    | 
    | % Signals 1&2 valid
    | 
    | num = 2;
    | select(1)=1;
    | select(2)=2;
    | 
    | function aFcnTruthTableAction_3()
    | 
    | % Signals 1&3 valid
    | 
    | num = 2;
    | select(1)=1;
    | select(2)=3;
    | 
    | function aFcnTruthTableAction_4()
    | 
    | % Signals 2&3 valid
    | 
    | num = 2;
    | select(1)=2;
    | select(2)=3;
    | 
    | function aFcnTruthTableAction_5()
    | 
    | % Signal 1 valid
    | 
    | num = 1;
    | select(1)=1;
    | select(2)=0;
    | 
    | function aFcnTruthTableAction_6()
    | 
    | % Signal 2 valid
    | 
    | num = 1;
    | select(1)=2;
    | select(2)=0;
    | 
    | function aFcnTruthTableAction_7()
    | 
    | % Signal 3 valid
    | 
    | num = 1;
    | select(1)=3;
    | select(2)=0;
    | 
    | function None()
    | 
    | % no signals valid
    | 
    | num = 0;

== stateflow chart CockpitDisplayLib/Warnings ==
  state FlightPhases [parallel]
    settings: executionOrder=1
    state EnginesOff
      entry, during:
      FlightMode = 0;
    state PushbackAndTaxi
      entry, during:
      FlightMode = 1;
    state TakeoffCruiseDescent
      entry, during:
      FlightMode = 2;
    state Land
      entry, during:
      FlightMode = 3;
    (default) -> EnginesOff
    EnginesOff -> PushbackAndTaxi : % start electric power
        | [Engine_Mode == 2]
    PushbackAndTaxi -> TakeoffCruiseDescent : % speed greater than 100 knots
        | [PFD.AirSpeed>100*1.8]
    TakeoffCruiseDescent -> Land : % speed less than 100 knots
        | [PFD.AirSpeed<100*1.8]
  state ComponentModes [parallel]
    settings: executionOrder=2
    state Temp [parallel]
      settings: executionOrder=2
    state OilP [parallel]
      settings: executionOrder=4
    state RPM [parallel]
      settings: executionOrder=1
    state Fuel [parallel]
      settings: executionOrder=3
    state Hyd [parallel]
      settings: executionOrder=5
    state APU [parallel]
      settings: executionOrder=6
    state CabinPressure [parallel]
      settings: executionOrder=7
    state LandingGear [parallel]
      settings: executionOrder=8
  state WarningsComputation [parallel]
    settings: executionOrder=3
    state Phase1
      entry,during: output_msgID = calcMsgID();
      state msgID = calcMsgID [function]
        note: Conditions to Check for
            | 5	'ENG STARTING                  '
            | 11	'APU FIRE                      '
            | 12	'APU STATUS.... OK             '
            | 41	'LANDING GEAR OFF              '
            | 42	'LANDING GEAR ON               '
            | 43	'LANDING GEAR RETRACTING       '
            | 44	'LANDING GEAR ERROR            '
        (default) -> (junction 1162) : {id = 1;msgID = zeros(10,1);}
        (junction 1162) -> (junction 1163) [order 1] : [RPMProblem == 0]
        (junction 1162) -> (junction 1164) [order 2] : {msgID(id) = 12;id = id + 1;}
        (junction 1163) -> (junction 1165) : {msgID(id) = 5; id = id + 1;}
        (junction 1165) -> (junction 1164)
        (junction 1164) -> (junction 1166)
        (junction 1166) -> (junction 1167) [order 1] : [APUProblem == 1]
        (junction 1166) -> (junction 1168) [order 2]
        (junction 1167) -> (junction 1169) : {msgID(id) = 11;id = id + 1;}
        (junction 1169) -> (junction 1168)
        (junction 1168) -> (junction 1170)
        (junction 1170) -> (junction 1171) [order 1] : [LandingGearMode == 0]
        (junction 1170) -> (junction 1172) [order 2]
        (junction 1171) -> (junction 1182) : {msgID(id) = 41;id = id + 1;}
        (junction 1172) -> (junction 1173) [order 1] : [LandingGearMode == 1]
        (junction 1172) -> (junction 1593) [order 2]
        (junction 1173) -> (junction 1181) : {msgID(id) = 42;id = id + 1;}
        (junction 1593) -> (junction 1595) [order 1] : [LandingGearMode == 2]
        (junction 1593) -> (junction 1174) [order 2]
        (junction 1595) -> (junction 1591) : {msgID(id) = 45;id = id + 1;}
        (junction 1174) -> (junction 1175) [order 1] : [LandingGearMode == 3]
        (junction 1174) -> (junction 1176) [order 2]
        (junction 1175) -> (junction 1180) : {msgID(id) = 43;id = id + 1;}
        (junction 1176) -> (junction 1177) [order 1] : [LandingGearMode == 4]
        (junction 1176) -> (junction 1178) [order 2]
        (junction 1177) -> (junction 1179) : {msgID(id) = 44;id = id + 1;}
        (junction 1179) -> (junction 1178)
        (junction 1180) -> (junction 1179)
        (junction 1591) -> (junction 1180)
        (junction 1181) -> (junction 1591)
        (junction 1182) -> (junction 1181)
    state Phase2
      entry, during: output_msgID = calcMsgID();
      state msgID = calcMsgID [function]
        note: 51	'FUEL QUANTITY LOW             '
            | 52	'FUEL PRESSURE LOW             '
            | 3	'ENG 1(2) OIL LO PR            '
            | 4	'ENG OIL PRE.... OK            '
            | 31	'HYD PRESSURE LOW              '
            | 32	'HYD PRESSURE.... OK           '
            | 41	'LANDING GEAR OFF              '
            | 42	'LANDING GEAR ON               '
            | 43	'LANDING GEAR RETRACTING       '
            | 44	'LANDING GEAR ERROR            '
            | 6	'ENG 1 (2)       FAULT         '
            | 2	'ENG STATUS.... OK             '
            | 11	'APU FIRE                      '
        (default) -> (junction 1214) : {id = 1;msgID = zeros(10,1);}
        (junction 1214) -> (junction 1215) [order 1] : [FuelQProblem == 1]
        (junction 1214) -> (junction 1443) [order 2]
        (junction 1215) -> (junction 1442) : {msgID(id) = 51; id = id + 1;}
        (junction 1442) -> (junction 1443)
        (junction 1443) -> (junction 1216)
        (junction 1216) -> (junction 1217) [order 1] : [FuelPProblem == 1]
        (junction 1216) -> (junction 1438) [order 2]
        (junction 1217) -> (junction 1440) : {msgID(id) = 52; id = id + 1;}
        (junction 1440) -> (junction 1438)
        (junction 1438) -> (junction 1218)
        (junction 1218) -> (junction 1219) [order 1] : [OilPProblem == 1]
        (junction 1218) -> (junction 1435) [order 2] : {msgID(id) = 4;id = id + 1;}
        (junction 1219) -> (junction 1434) : {msgID(id) = 3;id = id + 1;}
        (junction 1434) -> (junction 1435)
        (junction 1435) -> (junction 1220)
        (junction 1220) -> (junction 1221) [order 1] : [HydProblem == 1]
        (junction 1220) -> (junction 1419) [order 2] : {msgID(id) = 32;id = id + 1;}
        (junction 1221) -> (junction 1420) : {msgID(id) = 31;id = id + 1;}
        (junction 1420) -> (junction 1419)
        (junction 1419) -> (junction 1634)
        (junction 1634) -> (junction 1633) [order 1] : [LandingGearMode == 0]
        (junction 1634) -> (junction 1627) [order 2]
        (junction 1633) -> (junction 1600) : {msgID(id) = 41;id = id + 1;}
        (junction 1627) -> (junction 1621) [order 1] : [LandingGearMode == 1]
        (junction 1627) -> (junction 1625) [order 2]
        (junction 1621) -> (junction 1604) : {msgID(id) = 42;id = id + 1;}
        (junction 1625) -> (junction 1619) [order 1] : [LandingGearMode == 2]
        (junction 1625) -> (junction 1623) [order 2]
        (junction 1619) -> (junction 1606) : {msgID(id) = 45;id = id + 1;}
        (junction 1623) -> (junction 1612) [order 1] : [LandingGearMode == 3]
        (junction 1623) -> (junction 1626) [order 2]
        (junction 1612) -> (junction 1610) : {msgID(id) = 43;id = id + 1;}
        (junction 1626) -> (junction 1616) [order 1] : [LandingGearMode == 4]
        (junction 1626) -> (junction 1624) [order 2]
        (junction 1616) -> (junction 1615) : {msgID(id) = 44;id = id + 1;}
        (junction 1615) -> (junction 1624)
        (junction 1610) -> (junction 1615)
        (junction 1606) -> (junction 1610)
        (junction 1604) -> (junction 1606)
        (junction 1600) -> (junction 1604)
        (junction 1624) -> (junction 1235)
        (junction 1235) -> (junction 1236) [order 1] : [RPMProblem == 1]
        (junction 1235) -> (junction 1446) [order 2] : {msgID(id) = 2;id = id + 1;}
        (junction 1236) -> (junction 1449) : {msgID(id) = 6;id = id + 1;}
        (junction 1449) -> (junction 1446)
        (junction 1446) -> (junction 1237)
        (junction 1237) -> (junction 1238) [order 1] : [APUProblem == 1]
        (junction 1237) -> (junction 1239) [order 2]
        (junction 1238) -> (junction 1452) : {msgID(id) = 11;id = id + 1;}
        (junction 1452) -> (junction 1239)
    state Phase3
      entry, during: output_msgID = calcMsgID();
      state msgID = calcMsgID [function]
        note: 6	'ENG 1 (2) FAULT               '
            | 2	'ENG STATUS.... OK             '
            | 3	'ENG 1(2) OIL LO PR            '
            | 4	'ENG OIL PRE.... OK            '
            | 31	'HYD PRESSURE LOW              '
            | 32	'HYD PRESSURE.... OK           '
            | 11	'APU FIRE                      '
            | 51	'FUEL QUANTITY LOW             '
            | 52	'FUEL PRESSURE LOW             '
            | 41	'LANDING GEAR OFF              '
            | 42	'LANDING GEAR ON               '
            | 43	'LANDING GEAR RETRACTING       '
            | 44	'LANDING GEAR ERROR            '
            | 21	'CABIN PRESSURE LOW            '
            | 22	'CABIN PRESSURE.... OK         '
        (default) -> (junction 1280) : {id = 1;msgID = zeros(10,1);}
        (junction 1280) -> (junction 1281) [order 1] : [RPMProblem == 1]
        (junction 1280) -> (junction 1456) [order 2] : {msgID(id) = 2;id = id + 1;}
        (junction 1281) -> (junction 1455) : {msgID(id) = 6; id = id + 1;}
        (junction 1455) -> (junction 1456)
        (junction 1456) -> (junction 1282)
        (junction 1282) -> (junction 1283) [order 1] : [OilPProblem == 1]
        (junction 1282) -> (junction 1459) [order 2] : {msgID(id) = 4;id = id + 1;}
        (junction 1283) -> (junction 1460) : {msgID(id) = 3;id = id + 1;}
        (junction 1460) -> (junction 1459)
        (junction 1459) -> (junction 1284)
        (junction 1284) -> (junction 1285) [order 1] : [HydProblem == 1]
        (junction 1284) -> (junction 1463) [order 2] : {msgID(id) = 32;id = id + 1;}
        (junction 1285) -> (junction 1464) : {msgID(id) = 31;id = id + 1;}
        (junction 1464) -> (junction 1463)
        (junction 1463) -> (junction 1286)
        (junction 1286) -> (junction 1287) [order 1] : [APUProblem == 1]
        (junction 1286) -> (junction 1467) [order 2]
        (junction 1287) -> (junction 1468) : {msgID(id) = 11;id = id + 1;}
        (junction 1468) -> (junction 1467)
        (junction 1467) -> (junction 1288)
        (junction 1288) -> (junction 1289) [order 1] : [FuelQProblem == 1]
        (junction 1288) -> (junction 1471) [order 2]
        (junction 1289) -> (junction 1472) : {msgID(id) = 51;id = id + 1;}
        (junction 1472) -> (junction 1471)
        (junction 1471) -> (junction 1290)
        (junction 1290) -> (junction 1291) [order 1] : [FuelPProblem == 1]
        (junction 1290) -> (junction 1475) [order 2]
        (junction 1291) -> (junction 1476) : {msgID(id) = 52;id = id + 1;}
        (junction 1476) -> (junction 1475)
        (junction 1475) -> (junction 1292)
        (junction 1292) -> (junction 1293) [order 1] : [CabinPProblem == 1]
        (junction 1292) -> (junction 1294) [order 2] : {msgID(id) = 22;id = id + 1;}
        (junction 1293) -> (junction 1480) : {msgID(id) = 21;id = id + 1;}
        (junction 1480) -> (junction 1294)
        (junction 1294) -> (junction 1670)
        (junction 1670) -> (junction 1669) [order 1] : [LandingGearMode == 0]
        (junction 1670) -> (junction 1663) [order 2]
        (junction 1669) -> (junction 1636) : {msgID(id) = 41;id = id + 1;}
        (junction 1663) -> (junction 1657) [order 1] : [LandingGearMode == 1]
        (junction 1663) -> (junction 1661) [order 2]
        (junction 1657) -> (junction 1640) : {msgID(id) = 42;id = id + 1;}
        (junction 1661) -> (junction 1655) [order 1] : [LandingGearMode == 2]
        (junction 1661) -> (junction 1659) [order 2]
        (junction 1655) -> (junction 1642) : {msgID(id) = 45;id = id + 1;}
        (junction 1659) -> (junction 1648) [order 1] : [LandingGearMode == 3]
        (junction 1659) -> (junction 1662) [order 2]
        (junction 1648) -> (junction 1646) : {msgID(id) = 43;id = id + 1;}
        (junction 1662) -> (junction 1652) [order 1] : [LandingGearMode == 4]
        (junction 1662) -> (junction 1660) [order 2]
        (junction 1652) -> (junction 1651) : {msgID(id) = 44;id = id + 1;}
        (junction 1651) -> (junction 1660)
        (junction 1646) -> (junction 1651)
        (junction 1642) -> (junction 1646)
        (junction 1640) -> (junction 1642)
        (junction 1636) -> (junction 1640)
    state Phase4
      entry, during: output_msgID = calcMsgID();
      state msgID = calcMsgID [function]
        note: 52	'FUEL PRESSURE LOW             '
            | 3	'ENG 1(2) OIL LO PR            '
            | 4	'ENG OIL PRE.... OK            '
            | 31	'HYD PRESSURE LOW              '
            | 41	'LANDING GEAR OFF              '
            | 42	'LANDING GEAR ON               '
            | 43	'LANDING GEAR RETRACTING       '
            | 44	'LANDING GEAR ERROR            '
            | 6	'ENG 1 (2) FAULT               '
        (default) -> (junction 1351) : {id = 1;msgID = zeros(10,1);}
        (junction 1351) -> (junction 1352) [order 1] : [FuelPProblem == 1]
        (junction 1351) -> (junction 1482) [order 2]
        (junction 1352) -> (junction 1483) : {msgID(id) = 52; id = id + 1;}
        (junction 1483) -> (junction 1482)
        (junction 1482) -> (junction 1353)
        (junction 1353) -> (junction 1354) [order 1] : [OilPProblem == 1]
        (junction 1353) -> (junction 1486) [order 2] : {msgID(id) = 4;id = id + 1;}
        (junction 1354) -> (junction 1488) : {msgID(id) = 3;id = id + 1;}
        (junction 1488) -> (junction 1486)
        (junction 1486) -> (junction 1355)
        (junction 1355) -> (junction 1356) [order 1] : [HydProblem == 1]
        (junction 1355) -> (junction 1357) [order 2]
        (junction 1356) -> (junction 1490) : {msgID(id) = 31;id = id + 1;}
        (junction 1490) -> (junction 1357)
        (junction 1357) -> (junction 1706)
        (junction 1706) -> (junction 1705) [order 1] : [LandingGearMode == 0]
        (junction 1706) -> (junction 1699) [order 2]
        (junction 1705) -> (junction 1672) : {msgID(id) = 41;id = id + 1;}
        (junction 1699) -> (junction 1693) [order 1] : [LandingGearMode == 1]
        (junction 1699) -> (junction 1697) [order 2]
        (junction 1693) -> (junction 1676) : {msgID(id) = 42;id = id + 1;}
        (junction 1697) -> (junction 1691) [order 1] : [LandingGearMode == 2]
        (junction 1697) -> (junction 1695) [order 2]
        (junction 1691) -> (junction 1678) : {msgID(id) = 45;id = id + 1;}
        (junction 1695) -> (junction 1684) [order 1] : [LandingGearMode == 3]
        (junction 1695) -> (junction 1698) [order 2]
        (junction 1684) -> (junction 1682) : {msgID(id) = 43;id = id + 1;}
        (junction 1698) -> (junction 1688) [order 1] : [LandingGearMode == 4]
        (junction 1698) -> (junction 1696) [order 2]
        (junction 1688) -> (junction 1687) : {msgID(id) = 44;id = id + 1;}
        (junction 1687) -> (junction 1696)
        (junction 1682) -> (junction 1687)
        (junction 1678) -> (junction 1682)
        (junction 1676) -> (junction 1678)
        (junction 1672) -> (junction 1676)
        (junction 1696) -> (junction 1371)
        (junction 1371) -> (junction 1372) [order 1] : [RPMProblem == 1]
        (junction 1372) -> (junction 1493) : {msgID(id) = 6;id = id + 1;}
        (junction 1371) -> (junction 1373) [order 2]
        (junction 1493) -> (junction 1373)
    (default) -> Phase1
    Phase1 -> Phase2 : % move from EnginesOff to
        | % PushbackAndTaxi mode
        | [FlightMode == 1]
    Phase2 -> Phase3 : % move from PushbackAndTaxi
        | % to TakeoffCruiseDescent mode
        | [FlightMode == 2 ]
    Phase3 -> Phase4 : % move from TakeoffCruiseDescent
        | % to Land mode
        | [FlightMode == 3]
  data: msgID function_output double; msgID function_output double; msgID function_output double; msgID function_output double; APUMode input; output_msgID output double size=[10 1]; Engine_Mode input double; PFD input Bus: FlightInputs; EngNFuel input Bus: EngineFuel_Bus; Misc input Bus: MiscData; RPMProblem output double size=1; TempProblem output double size=1; FuelPProblem output double size=1; FuelQProblem output double size=1; OilPProblem output double size=1; FlightMode data_store_memory size=1; APUProblem output double size=1; HydProblem output double size=1; CabinPProblem output double size=1; id local double size=1; LandingGearMode output double size=1

== stateflow chart CockpitDisplayLib/Warnings/ComponentModes.APU ==
  state Normal
    entry:
    APUProblem = 0;
  state EngineFire
    entry:
    APUProblem = 1;
  (default) -> Normal
  Normal -> EngineFire : [(FlightMode == 0 && APUMode == 3)||...
      | ((FlightMode == 1 && Misc.APUData < 0.5)||(FlightMode == 2 && Misc.APUData < 0.8))]
  EngineFire -> Normal : [~((FlightMode == 0 && APUMode == 3)||...
      | ((FlightMode == 1 ||FlightMode == 2) && Misc.APUData < 0.8))]
  data: APUMode input; Misc input Bus: MiscData; FlightMode data_store_memory size=1; APUProblem output double size=1

== stateflow chart CockpitDisplayLib/Warnings/ComponentModes.CabinPressure ==
  state Normal
    entry:
    CabinPProblem = 0;
  state CabinPressureLow
    entry:
    CabinPProblem = 1;
  (default) -> Normal
  Normal -> CabinPressureLow : [(FlightMode == 1||FlightMode == 2)...
      | && Misc.CabinPressure < 0.5]
  CabinPressureLow -> Normal : [~((FlightMode == 1||FlightMode == 2)...
      | && Misc.CabinPressure < 0.5)]
  data: Misc input Bus: MiscData; FlightMode data_store_memory size=1; CabinPProblem output double size=1

== stateflow chart CockpitDisplayLib/Warnings/ComponentModes.Hyd ==
  state Hyd
    state Normal
      entry:
      HydProblem = 0;
    state EngineFire
      entry:
      HydProblem = 1;
    (default) -> Normal
    EngineFire -> Normal : [~((FlightMode == 1 && Misc.HydraulicPressure < 500)|| ...
        | ((FlightMode == 2||FlightMode == 3)&& Misc.HydraulicPressure < 1500))] %psi
    Normal -> EngineFire : [(FlightMode == 1 && Misc.HydraulicPressure < 500)|| ...
        | ((FlightMode == 2||FlightMode == 3)...
        |  & Misc.HydraulicPressure < 1500)] %psi
  data: Misc input Bus: MiscData; FlightMode data_store_memory size=1; HydProblem output double size=1

== stateflow chart CockpitDisplayLib/Warnings/ComponentModes.OilP ==
  state Normal
    entry:
    OilPProblem = 0;
  state EngineOilLowPressure
    entry:
    OilPProblem = 1;
  (default) -> Normal
  Normal -> EngineOilLowPressure : [(FlightMode == 1 && EngNFuel.oilpressure < 1000)||...
      | ((FlightMode == 2 || FlightMode == 3)...
      | && EngNFuel.oilpressure < 2000)] %psi
  EngineOilLowPressure -> Normal : [~((FlightMode == 1 && EngNFuel.oilpressure < 1000)||...
      | ((FlightMode == 2 || FlightMode == 3)...
      | && EngNFuel.oilpressure < 2000))] %psi
  data: EngNFuel input Bus: EngineFuel_Bus; OilPProblem output double size=1; FlightMode data_store_memory
